simulink model "test6"  (R2024a)
settings: Solver=FixedStepAuto  StartTime=0.0  StopTime=300  RelTol=1e-3  EnableMultiTasking=on
libraries: arduinolib x3
settings Model: ExtModeTrigDuration=2  Creator=ADMIN  LastModifiedBy=thanh
settings OptimizationCC: EnhancedBackFolding=on  PassReuseOutputArgsThreshold=0  MaxStackSize=64  OptimizeBlockOrder=speed  DifferentSizesBufferReuse=on  OptimizationCustomize=off
settings DebuggingCC: ParameterTunabilityLossMsg=error
settings HardwareCC: ProdBitPerInt=16  ProdBitPerPointer=16  ProdBitPerSizeT=16  ProdBitPerPtrDiffT=16  ProdLargestAtomicFloat=None  ProdWordSize=8  ProdHWDeviceType=Atmel->AVR
settings SFSimCC: MATLABDynamicMemAlloc=off
settings RTWCC: Description=Embedded Coder  SystemTargetFile=ert.tlc  HardwareBoard=Arduino Uno  TemplateMakefile=ert_default_tmf  Toolchain=Arduino AVR  BuildConfiguration=Faster Runs  GPUComputeCapability=3.5
settings CodeAppCC: ForceParamTrailComments=on  OperatorAnnotations=on
settings ERTTargetCC: ERTCustomFileBanners=off  SupportContinuousTime=on  SupportNonInlinedSFcns=on  RemoveResetFunc=off  SupportVariableSizeSignals=on  ModelStepFunctionPrototypeControlCompliant=off  ExtModeTransport=3  ExtModeStaticAlloc=on  ExtModeAutomaticAllocSize=off  ExtModeStaticAllocSize=250  ExtModeMexFile=ext_xcp  ExtModeIntrfLevel=Level2 - Open

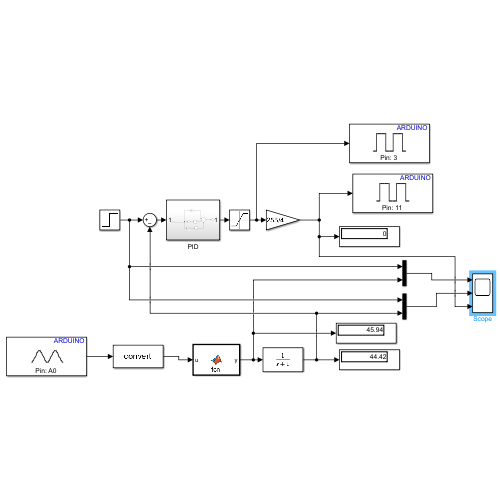
[thumbnail: Simulink's stored preview of the top-level diagram]
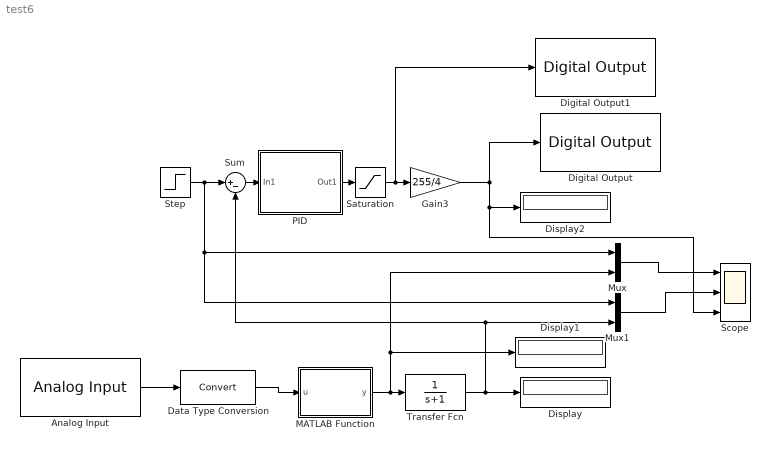
== system test6 ==
  Analog Input : arduinolib/Analog Input  pinNumber=0  ReadResultsOnly=off  ConversionTriggerSource=Software  ExternalTriggerType=uint32( 0 )  OutputDataType=uint16  EnableConversionCompleteNotify=off  EnableOuputStatus=off  SampleTime=-1  blockPlatform=arduino
  Data Type Conversion : DataTypeConversion  SaturateOnIntegerOverflow=off  RndMeth=Floor
  Digital Output : arduinolib/Digital Output  pinNumber=11  Direction=output  blockPlatform=arduino
  Digital Output1 : arduinolib/Digital Output  pinNumber=3  Direction=output  blockPlatform=arduino
  Display : Display
  Display1 : Display
  Display2 : Display
  Gain3 : Gain  Gain=255/4
  MATLAB Function : MATLAB Function  TreatAsAtomicUnit=on
  Mux : Mux  Inputs=2
  Mux1 : Mux  Inputs=2
  PID : Subsystem
  Saturation : Saturate  UpperLimit=255  LowerLimit=0
  Scope : Scope  NumInputPorts=3
  Step : Step  After=45  SampleTime=0.5
  Sum : Sum  Inputs=|+-
  Transfer Fcn : TransferFcn  Denominator=[1 1]
  wires:
  Step/1 -> Mux/1, Mux1/1, Sum/1
  Saturation/1 -> Digital Output1/1, Gain3/1
  Sum/1 -> PID/1(In1)
  PID/1(Out1) -> Saturation/1
  MATLAB Function/1(y) -> Transfer Fcn/1, Display1/1, Mux/2
  Gain3/1 -> Digital Output/1, Display2/1, Scope/3
  Transfer Fcn/1 -> Mux1/2, Sum/2, Display/1
  Mux/1 -> Scope/1
  Mux1/1 -> Scope/2
  Data Type Conversion/1 -> MATLAB Function/1(u)
  Analog Input/1 -> Data Type Conversion/1

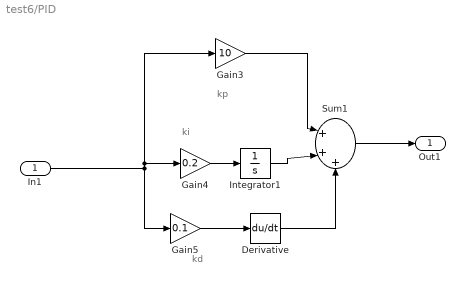
== system test6/PID ==
  note: kp
  note: ki
  note: kd
  In1 : Inport
  Derivative : Derivative
  Gain3 : Gain  Gain=10
  Gain4 : Gain  Gain=0.2
  Gain5 : Gain  Gain=0.1
  Integrator1 : Integrator
  Sum1 : Sum  Inputs=|+++
  Out1 : Outport
  wires:
  Gain5/1 -> Derivative/1
  Sum1/1 -> Out1/1
  Derivative/1 -> Sum1/3
  In1/1 -> Gain3/1, Gain4/1, Gain5/1
  Gain3/1 -> Sum1/1
  Integrator1/1 -> Sum1/2
  Gain4/1 -> Integrator1/1

== matlab function test6/MATLAB Function ==
  data: u input; y output
function y = fcn(u)

y = (u*5/1023)*100;
